simulink library "plant_cl"  (R2018a)
settings: Solver=VariableStepAuto  StartTime=0.0  StopTime=10.0  RelTol=1e-3
undefined symbols (not defined in the file or in its folder): env, faults, p, plant
libraries: lowLevel x29, controllerComponents x1
settings Model: Creator=mitch  LastModifiedBy=mitch

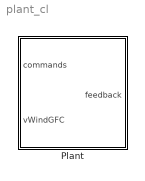
== system plant_cl ==
  Plant : Subsystem

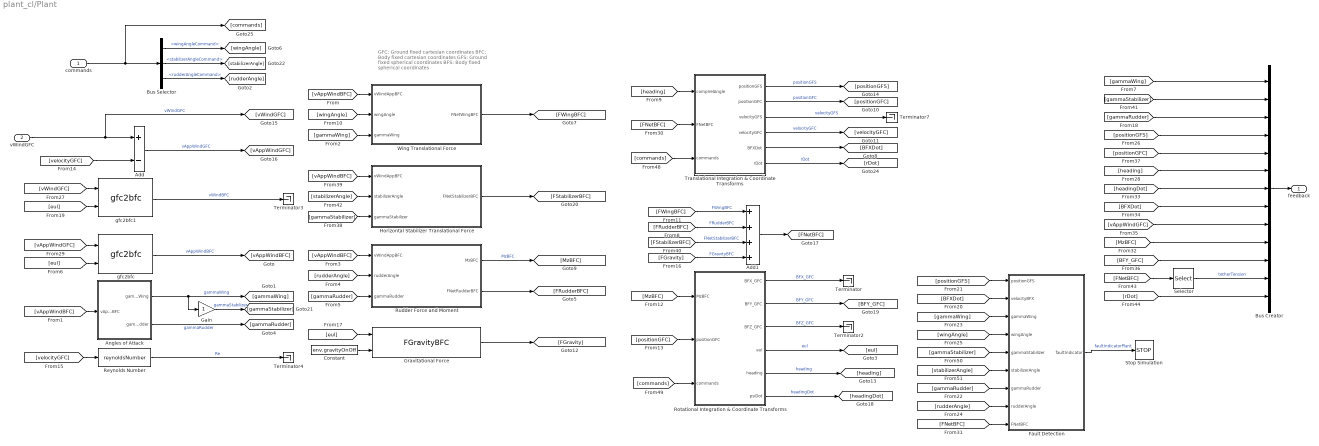
== system plant_cl/Plant ==
  note: GFC: Ground fixed cartesian coordinates
      | BFC:  Body fixed cartesian coordinates
      | GFS: Ground fixed spherical coordinates
      | BFS: Body fixed spherical coordinates
  commands : Inport  OutDataTypeStr=Bus: busControllerOutput
  vWindGFC : Inport  Port=2
  Add : Sum  Inputs=+-
  Add1 : Sum  Inputs=++++
  Angles of Attack : Subsystem
  Bus Selector : BusSelector  OutputSignals=wingAngleCommand,stabilizerAngleCommand,rudderAngleCommand
  Bus Creator : BusCreator  Inputs=13  OutDataTypeStr=Bus: busPlantFeedback
  Constant : Constant  Value=env.gravityOnOff
  Fault Detection : Subsystem
  Gain : Gain
  Gravitational Force : lowLevel/FGravityBFC
  Horizontal Stabilizer Translational Force : Subsystem
  Reynolds Number : lowLevel/reynoldsNumber
  Rotational Integration & Coordinate Transforms : Subsystem
  Rudder Force and Moment : Subsystem
  Selector : Selector  InputPortWidth=3  IndexOptions=Index vector (dialog)  Indices=3  OutputSizes=1
  Stop Simulation : Stop
  Terminator{,2..4,7} (5 alike) : Terminator
  Translational Integration & Coordinate Transforms : Subsystem
  Wing Translational Force : Subsystem
  gfc2bfc : lowLevel/gfc2bfc
  gfc2bfc1 : lowLevel/gfc2bfc
  feedback : Outport  OutDataTypeStr=Bus: busPlantFeedback
  wires:
  vWindGFC/1 -> [vWindGFC], Add/1  "vWindGFC"
  [vAppWindBFC] -> Angles of Attack/1(vAppWindBFC)
  Angles of Attack/1(gammaWing) -> Gain/1, [gammaWing]  "gammaWing"
  [vAppWindBFC] -> Wing Translational Force/1(vWindAppBFC)
  Add/1 -> [vAppWindGFC]  "vAppWindGFC"
  [vAppWindBFC] -> Rudder Force and Moment/1(vWindAppBFC)
  [rudderAngle] -> Rudder Force and Moment/2(rudderAngle)
  Translational Integration & Coordinate Transforms/2(positionGFC) -> [positionGFC]  "positionGFC"
  Rudder Force and Moment/2(FNetRudderBFC) -> [FRudderBFC]
  [gammaWing] -> Wing Translational Force/3(gammaWing)
  [heading] -> Translational Integration & Coordinate Transforms/1(compVelAngle)
  Angles of Attack/2(gammaRudder) -> [gammaRudder]  "gammaRudder"
  [gammaRudder] -> Rudder Force and Moment/3(gammaRudder)
  Wing Translational Force/1(FNetWingBFC) -> [FWingBFC]
  [wingAngle] -> Wing Translational Force/2(wingAngle)
  [FNetBFC] -> Translational Integration & Coordinate Transforms/2(FNetBFC)
  Rudder Force and Moment/1(MzBFC) -> [MzBFC]  "MzBFC"
  [MzBFC] -> Rotational Integration & Coordinate Transforms/1(MzBFC)
  [positionGFC] -> Rotational Integration & Coordinate Transforms/2(positionGFC)
  Rotational Integration & Coordinate Transforms/4(eul) -> [eul]  "eul"
  Rotational Integration & Coordinate Transforms/1(BFX_GFC) -> Terminator/1  "BFX_GFC"
  Rotational Integration & Coordinate Transforms/2(BFY_GFC) -> [BFY_GFC]  "BFY_GFC"
  Rotational Integration & Coordinate Transforms/3(BFZ_GFC) -> Terminator2/1  "BFZ_GFC"
  Translational Integration & Coordinate Transforms/4(velocityGFC) -> [velocityGFC]  "velocityGFC"
  [velocityGFC] -> Add/2
  [velocityGFC] -> Reynolds Number/1
  Reynolds Number/1 -> Terminator4/1  "Re"
  Gravitational Force/1 -> [FGravity]
  [eul] -> Gravitational Force/1
  Translational Integration & Coordinate Transforms/1(positionGFS) -> [positionGFS]  "positionGFS"
  Translational Integration & Coordinate Transforms/3(velocityGFS) -> Terminator7/1  "velocityGFS"
  [eul] -> gfc2bfc1/2
  gfc2bfc1/1 -> Terminator3/1  "vWindBFC"
  Rotational Integration & Coordinate Transforms/5(heading) -> [heading]  "heading"
  Constant/1 -> Gravitational Force/2
  Translational Integration & Coordinate Transforms/5(BFXDot) -> [BFXDot]
  [BFXDot] -> Fault Detection/2(velocityBFX)
  [positionGFS] -> Fault Detection/1(positionGFS)
  Fault Detection/1(faultIndicator) -> Stop Simulation/1  "faultIndicatorPlant"
  [gammaRudder] -> Fault Detection/7(gammaRudder)
  [gammaWing] -> Fault Detection/3(gammaWing)
  [rudderAngle] -> Fault Detection/8(rudderAngle)
  [wingAngle] -> Fault Detection/4(wingAngle)
  [vWindGFC] -> gfc2bfc1/1
  gfc2bfc/1 -> [vAppWindBFC]  "vAppWindBFC"
  [eul] -> gfc2bfc/2
  [vAppWindGFC] -> gfc2bfc/1
  [FWingBFC] -> Add1/1  "FWingBFC"
  [FRudderBFC] -> Add1/2  "FRudderBFC"
  Add1/1 -> [FNetBFC]
  [FNetBFC] -> Fault Detection/9(FNetBFC)
  commands/1 -> [commands], Bus Selector/1
  Bus Selector/1 -> [wingAngle]  "<wingAngleCommand>"
  Bus Selector/3 -> [rudderAngle]  "<rudderAngleCommand>"
  Bus Creator/1 -> feedback/1
  Rotational Integration & Coordinate Transforms/6(psiDot) -> [headingDot]  "headingDot"
  [gammaStabilizer] -> Horizontal Stabilizer Translational Force/3(gammaStabilizer)
  [vAppWindBFC] -> Horizontal Stabilizer Translational Force/1(vWindAppBFC)
  Horizontal Stabilizer Translational Force/1(FNetStabilizerBFC) -> [FStabilizerBFC]
  [FStabilizerBFC] -> Add1/3  "FNetStabilizerBFC"
  [FGravity] -> Add1/4  "FGravityBFC"
  Translational Integration & Coordinate Transforms/6(rDot) -> [rDot]  "rDot"
  [commands] -> Translational Integration & Coordinate Transforms/3(commands)
  [commands] -> Rotational Integration & Coordinate Transforms/3(commands)
  [stabilizerAngle] -> Horizontal Stabilizer Translational Force/2(stabilizerAngle)
  Bus Selector/2 -> [stabilizerAngle]  "<stabilizerAngleCommand>"
  [gammaStabilizer] -> Fault Detection/5(gammaStabilizer)
  [stabilizerAngle] -> Fault Detection/6(stabilizerAngle)
  [gammaWing] -> Bus Creator/1
  [gammaRudder] -> Bus Creator/3
  [rDot] -> Bus Creator/13
  Selector/1 -> Bus Creator/12  "tetherTension"
  [BFY_GFC] -> Bus Creator/11
  [MzBFC] -> Bus Creator/10
  [vAppWindGFC] -> Bus Creator/9
  [BFXDot] -> Bus Creator/8
  [headingDot] -> Bus Creator/7
  [heading] -> Bus Creator/6
  [positionGFC] -> Bus Creator/5
  [positionGFS] -> Bus Creator/4
  [gammaStabilizer] -> Bus Creator/2
  Gain/1 -> [gammaStabilizer]  "gammaStabilizer"
  [FNetBFC] -> Selector/1

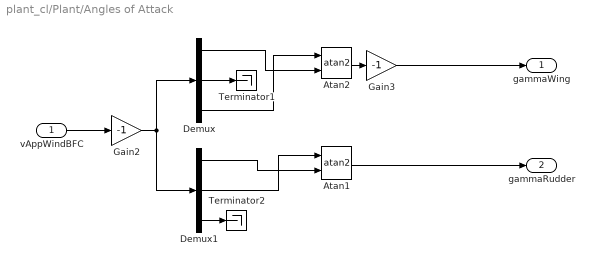
== system plant_cl/Plant/Angles of Attack ==
  vAppWindBFC : Inport
  Atan1 : Trigonometry  Operator=atan2
  Atan2 : Trigonometry  Operator=atan2
  Demux : Demux  Outputs=3
  Demux1 : Demux  Outputs=3
  Gain2 : Gain  Gain=-1
  Gain3 : Gain  Gain=-1
  Terminator1 : Terminator
  Terminator2 : Terminator
  gammaWing : Outport
  gammaRudder : Outport  Port=2
  wires:
  vAppWindBFC/1 -> Gain2/1
  Demux/1 -> Atan2/2
  Atan2/1 -> Gain3/1
  Demux/3 -> Atan2/1
  Demux/2 -> Terminator1/1
  Demux1/3 -> Terminator2/1
  Gain2/1 -> Demux1/1, Demux/1
  Atan1/1 -> gammaRudder/1
  Gain3/1 -> gammaWing/1
  Demux1/1 -> Atan1/2
  Demux1/2 -> Atan1/1

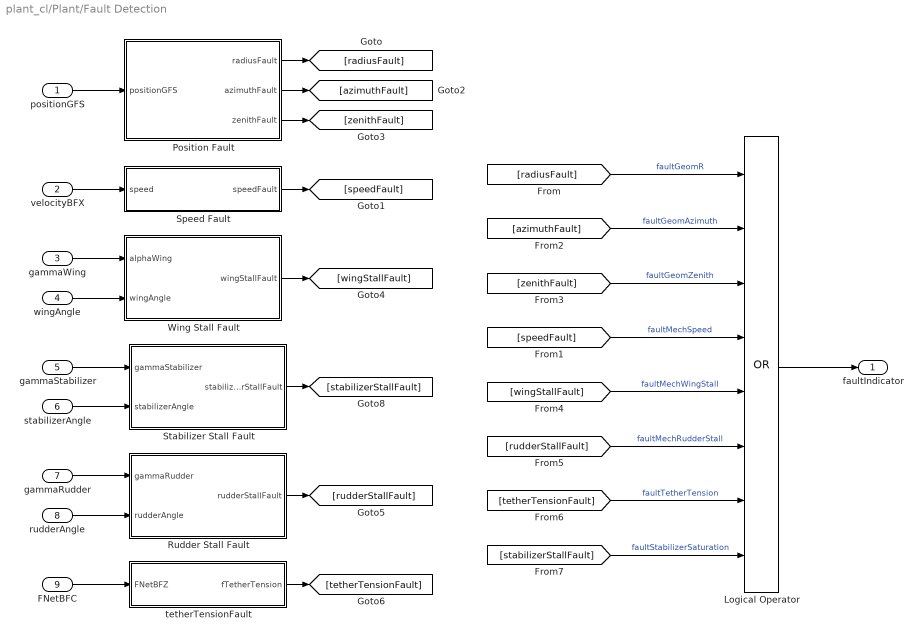
== system plant_cl/Plant/Fault Detection ==
  positionGFS : Inport
  velocityBFX : Inport  Port=2
  gammaWing : Inport  Port=3
  wingAngle : Inport  Port=4
  gammaStabilizer : Inport  Port=5
  stabilizerAngle : Inport  Port=6
  gammaRudder : Inport  Port=7
  rudderAngle : Inport  Port=8
  FNetBFC : Inport  Port=9
  Logical Operator : Logic  Operator=OR  Inputs=8  AllPortsSameDT=off  OutDataTypeStr=boolean
  Position Fault : Subsystem
  Rudder Stall Fault : Subsystem
  Speed Fault : Subsystem
  Stabilizer Stall Fault : Subsystem
  Wing Stall Fault : Subsystem
  tetherTensionFault : Subsystem
  faultIndicator : Outport
  wires:
  positionGFS/1 -> Position Fault/1(positionGFS)
  Logical Operator/1 -> faultIndicator/1
  Speed Fault/1(speedFault) -> [speedFault]
  velocityBFX/1 -> Speed Fault/1(speed)
  [radiusFault] -> Logical Operator/1  "faultGeomR"
  [speedFault] -> Logical Operator/4  "faultMechSpeed"
  [azimuthFault] -> Logical Operator/2  "faultGeomAzimuth"
  [zenithFault] -> Logical Operator/3  "faultGeomZenith"
  Wing Stall Fault/1(wingStallFault) -> [wingStallFault]
  gammaWing/1 -> Wing Stall Fault/1(alphaWing)
  gammaRudder/1 -> Rudder Stall Fault/1(gammaRudder)
  [wingStallFault] -> Logical Operator/5  "faultMechWingStall"
  [rudderStallFault] -> Logical Operator/6  "faultMechRudderStall"
  wingAngle/1 -> Wing Stall Fault/2(wingAngle)
  rudderAngle/1 -> Rudder Stall Fault/2(rudderAngle)
  Rudder Stall Fault/1(rudderStallFault) -> [rudderStallFault]
  Position Fault/1(radiusFault) -> [radiusFault]
  Position Fault/2(azimuthFault) -> [azimuthFault]
  Position Fault/3(zenithFault) -> [zenithFault]
  tetherTensionFault/1(fTetherTension) -> [tetherTensionFault]
  FNetBFC/1 -> tetherTensionFault/1(FNetBFZ)
  [tetherTensionFault] -> Logical Operator/7  "faultTetherTension"
  [stabilizerStallFault] -> Logical Operator/8  "faultStabilizerSaturation"
  gammaStabilizer/1 -> Stabilizer Stall Fault/1(gammaStabilizer)
  Stabilizer Stall Fault/1(stabilizerStallFault) -> [stabilizerStallFault]
  stabilizerAngle/1 -> Stabilizer Stall Fault/2(stabilizerAngle)

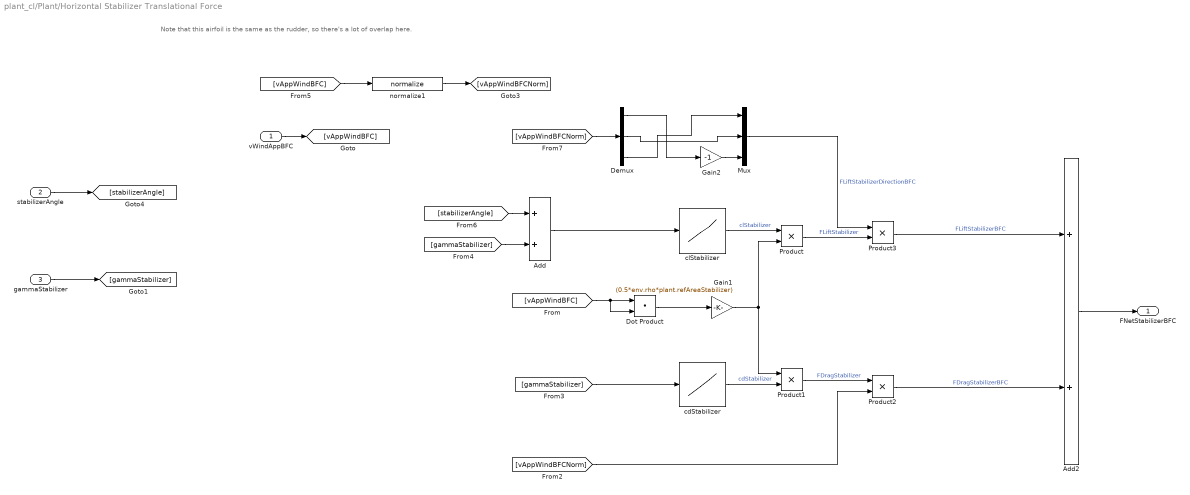
== system plant_cl/Plant/Horizontal Stabilizer Translational Force ==
  note: Note that this airfoil is the same as the rudder, so there's a lot of overlap here.
  vWindAppBFC : Inport
  stabilizerAngle : Inport  Port=2
  gammaStabilizer : Inport  Port=3
  Add : Sum
  Add2 : Sum
  Demux : Demux  Outputs=3
  Dot Product : DotProduct  InputSameDT=on  OutDataTypeStr=Inherit: Inherit via internal rule
  Gain1 : Gain  Gain=(0.5*env.rho*plant.refAreaStabilizer)
  Gain2 : Gain  Gain=-1
  Mux : Mux  Inputs=3
  Product{,1..3} (4 alike) : Product
  cdStabilizer : Lookup_n-D  NumberOfTableDimensions=1  BreakpointsForDimension1=plant.stabilizerTable.alpha  Table=plant.rudderTable.cd  ExtrapMethod=Clip  UseLastTableValue=on  InternalRulePriority=Speed  RndMeth=Simplest  InputSameDT=on
  clStabilizer : Lookup_n-D  NumberOfTableDimensions=1  BreakpointsForDimension1=plant.stabilizerTable.alpha  Table=plant.rudderTable.cl  ExtrapMethod=Clip  UseLastTableValue=on  InternalRulePriority=Speed  RndMeth=Simplest  InputSameDT=on
  normalize1 : lowLevel/normalize
  FNetStabilizerBFC : Outport
  wires:
  Product1/1 -> Product2/1  "FDragStabilizer"
  Product2/1 -> Add2/2  "FDragStabilizerBFC"
  Product/1 -> Product3/2  "FLiftStabilizer"
  Product3/1 -> Add2/1  "FLiftStabilizerBFC"
  Dot Product/1 -> Gain1/1
  clStabilizer/1 -> Product/1  "clStabilizer"
  [vAppWindBFC] -> Dot Product/1, Dot Product/2
  Gain1/1 -> Product/2, Product1/1
  cdStabilizer/1 -> Product1/2  "cdStabilizer"
  vWindAppBFC/1 -> [vAppWindBFC]
  Demux/2 -> Mux/2
  Demux/1 -> Gain2/1
  Mux/1 -> Product3/1  "FLiftStabilizerDirectionBFC"
  Demux/3 -> Mux/1
  [vAppWindBFC] -> normalize1/1
  normalize1/1 -> [vAppWindBFCNorm]
  [vAppWindBFCNorm] -> Demux/1
  [vAppWindBFCNorm] -> Product2/2
  Gain2/1 -> Mux/3
  [gammaStabilizer] -> cdStabilizer/1
  gammaStabilizer/1 -> [gammaStabilizer]
  Add2/1 -> FNetStabilizerBFC/1
  Add/1 -> clStabilizer/1
  [gammaStabilizer] -> Add/2
  stabilizerAngle/1 -> [stabilizerAngle]
  [stabilizerAngle] -> Add/1

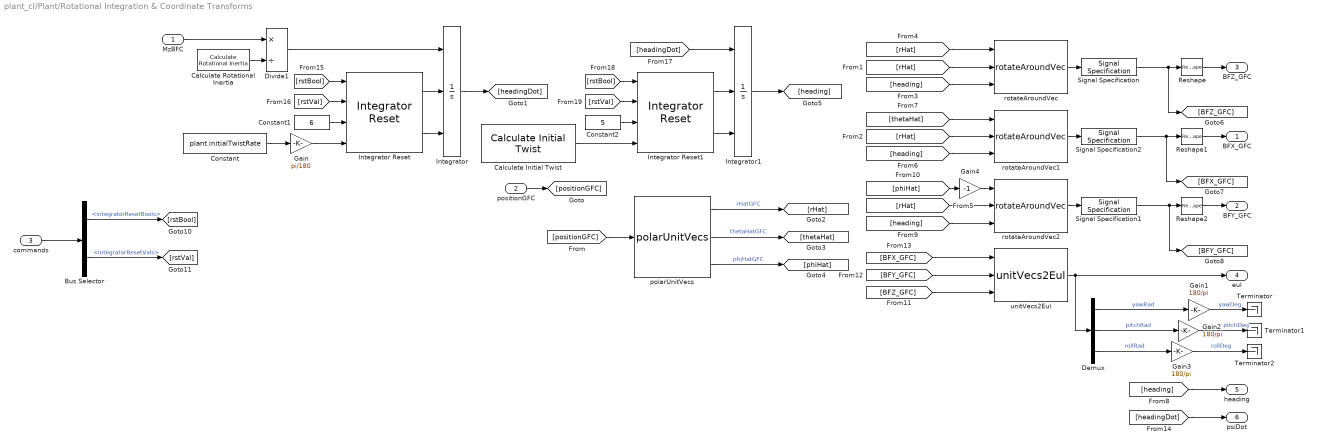
== system plant_cl/Plant/Rotational Integration & Coordinate Transforms ==
  MzBFC : Inport  PortDimensions=1
  positionGFC : Inport  Port=2
  commands : Inport  Port=3  OutDataTypeStr=Bus: busControllerOutput  PortDimensions=1
  Bus Selector : BusSelector  OutputSignals=integratorResetBools,integratorResetVals
  Calculate Rotational Inertia : lowLevel/Calculate Rotational Inertia
  Calculate Initial Twist : controllerComponents/Calculate Initial Twist
  Constant : Constant  Value=plant.initialTwistRate
  Constant1 : Constant  Value=6
  Constant2 : Constant  Value=5
  Demux : Demux  Outputs=3
  Divide1 : Product  Inputs=*/
  Gain : Gain  Gain=pi/180
  Gain1 : Gain  Gain=180/pi
  Gain2 : Gain  Gain=180/pi
  Gain3 : Gain  Gain=180/pi
  Gain4 : Gain  Gain=-1
  Integrator : Integrator  ExternalReset=rising  InitialConditionSource=external  InitialCondition=plant.initialTwistRate
  Integrator Reset : lowLevel/Integrator Reset
  Integrator Reset1 : lowLevel/Integrator Reset
  Integrator1 : Integrator  ExternalReset=rising  InitialConditionSource=external  InitialCondition=plant.initialTwist
  Reshape : Reshape  OutputDimensions=[3 1]
  Reshape1 : Reshape  OutputDimensions=[3 1]
  Reshape2 : Reshape  OutputDimensions=[3 1]
  Signal Specification : SignalSpecification  Dimensions=[1 3]
  Signal Specification1 : SignalSpecification  Dimensions=[1 3]
  Signal Specification2 : SignalSpecification  Dimensions=[1 3]
  Terminator : Terminator
  Terminator1 : Terminator
  Terminator2 : Terminator
  polarUnitVecs : lowLevel/polarUnitVecs
  rotateAroundVec : lowLevel/rotateAroundVec
  rotateAroundVec1 : lowLevel/rotateAroundVec
  rotateAroundVec2 : lowLevel/rotateAroundVec
  unitVecs2Eul : lowLevel/unitVecs2Eul
  BFX_GFC : Outport
  BFY_GFC : Outport  Port=2
  BFZ_GFC : Outport  Port=3
  eul : Outport  Port=4  PortDimensions=3
  heading : Outport  Port=5  PortDimensions=1
  psiDot : Outport  Port=6  PortDimensions=1
  wires:
  MzBFC/1 -> Divide1/1
  Integrator/1 -> [headingDot]
  positionGFC/1 -> [positionGFC]
  [positionGFC] -> polarUnitVecs/1
  polarUnitVecs/1 -> [rHat]  "rHatGFC"
  polarUnitVecs/2 -> [thetaHat]  "thetaHatGFC"
  polarUnitVecs/3 -> [phiHat]  "phiHatGFC"
  Integrator1/1 -> [heading]
  [heading] -> rotateAroundVec/3
  [rHat] -> rotateAroundVec/1
  [rHat] -> rotateAroundVec/2
  [thetaHat] -> rotateAroundVec1/1
  [heading] -> rotateAroundVec1/3
  [rHat] -> rotateAroundVec1/2
  [phiHat] -> Gain4/1
  [heading] -> rotateAroundVec2/3
  [rHat] -> rotateAroundVec2/2
  unitVecs2Eul/1 -> Demux/1, eul/1
  [BFZ_GFC] -> unitVecs2Eul/3
  [BFY_GFC] -> unitVecs2Eul/2
  [BFX_GFC] -> unitVecs2Eul/1
  Demux/3 -> Gain3/1  "rollRad"
  Demux/2 -> Gain2/1  "pitchRad"
  Demux/1 -> Gain1/1  "yawRad"
  Gain1/1 -> Terminator/1  "yawDeg"
  Gain2/1 -> Terminator1/1  "pitchDeg"
  Gain3/1 -> Terminator2/1  "rollDeg"
  Gain4/1 -> rotateAroundVec2/1
  rotateAroundVec/1 -> Signal Specification/1
  rotateAroundVec1/1 -> Signal Specification2/1
  rotateAroundVec2/1 -> Signal Specification1/1
  Signal Specification/1 -> Reshape/1, [BFZ_GFC]
  Signal Specification2/1 -> [BFX_GFC], Reshape1/1
  Signal Specification1/1 -> [BFY_GFC], Reshape2/1
  Reshape/1 -> BFZ_GFC/1
  Reshape1/1 -> BFX_GFC/1
  Reshape2/1 -> BFY_GFC/1
  [heading] -> heading/1
  [headingDot] -> psiDot/1
  Calculate Rotational Inertia/1 -> Divide1/2
  Divide1/1 -> Integrator/1
  Bus Selector/2 -> [rstVal]  "<integratorResetVals>"
  commands/1 -> Bus Selector/1
  Bus Selector/1 -> [rstBool]  "<integratorResetBools>"
  Integrator Reset1/1 -> Integrator1/2
  Integrator Reset1/2 -> Integrator1/3
  Integrator Reset/1 -> Integrator/2
  Integrator Reset/2 -> Integrator/3
  Constant/1 -> Gain/1
  [rstBool] -> Integrator Reset/1
  [rstVal] -> Integrator Reset/2
  Constant1/1 -> Integrator Reset/3
  Gain/1 -> Integrator Reset/4
  [headingDot] -> Integrator1/1
  [rstVal] -> Integrator Reset1/2
  Constant2/1 -> Integrator Reset1/3
  [rstBool] -> Integrator Reset1/1
  Calculate Initial Twist/1 -> Integrator Reset1/4

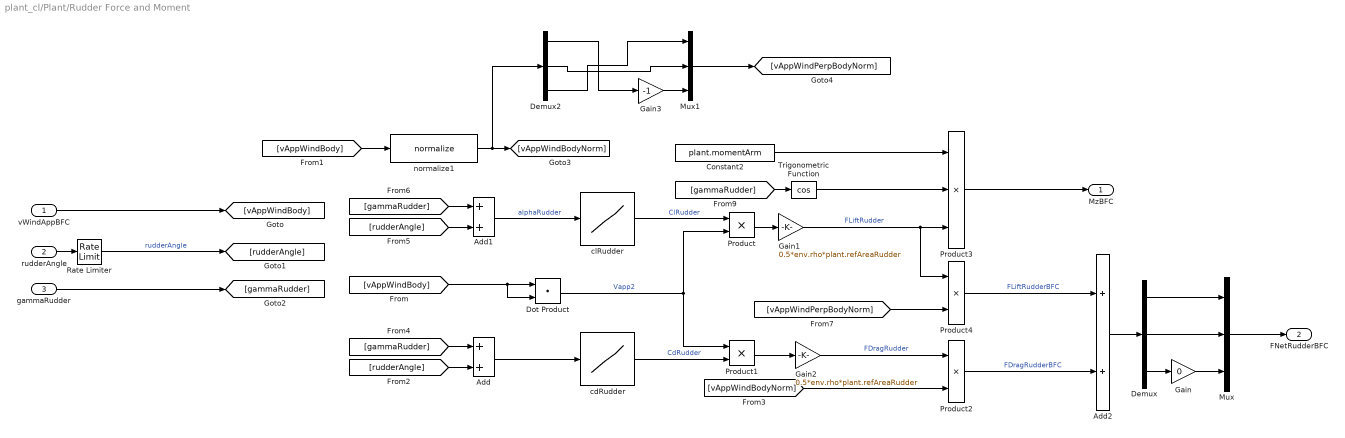
== system plant_cl/Plant/Rudder Force and Moment ==
  vWindAppBFC : Inport
  rudderAngle : Inport  Port=2
  gammaRudder : Inport  Port=3
  Add : Sum
  Add1 : Sum
  Add2 : Sum
  Constant2 : Constant  Value=plant.momentArm
  Demux : Demux  Outputs=3
  Demux2 : Demux  Outputs=3
  Dot Product : DotProduct  InputSameDT=on  OutDataTypeStr=Inherit: Inherit via internal rule
  Gain : Gain  Gain=0
  Gain1 : Gain  Gain=0.5*env.rho*plant.refAreaRudder
  Gain2 : Gain  Gain=0.5*env.rho*plant.refAreaRudder
  Gain3 : Gain  Gain=-1
  Mux : Mux  Inputs=3
  Mux1 : Mux  Inputs=3
  Product{,1..2,4} (4 alike) : Product
  Product3 : Product  Inputs=3
  Rate Limiter : RateLimiter  RisingSlewLimit=plant.rudderAngleRateLimit*pi/180  FallingSlewLimit=-plant.rudderAngleRateLimit*pi/180  SampleTimeMode=inherited
  Trigonometric Function : Trigonometry  Operator=cos
  cdRudder : Lookup_n-D  NumberOfTableDimensions=1  BreakpointsForDimension1=plant.rudderTable.alpha  Table=plant.rudderTable.cd  ExtrapMethod=Clip  UseLastTableValue=on  InternalRulePriority=Speed  RndMeth=Simplest  InputSameDT=on
  clRudder : Lookup_n-D  NumberOfTableDimensions=1  BreakpointsForDimension1=plant.rudderTable.alpha  Table=plant.rudderTable.cl  ExtrapMethod=Clip  UseLastTableValue=on  InternalRulePriority=Speed  RndMeth=Simplest  InputSameDT=on
  normalize1 : lowLevel/normalize
  MzBFC : Outport
  FNetRudderBFC : Outport  Port=2
  wires:
  clRudder/1 -> Product/1  "ClRudder"
  [vAppWindBody] -> Dot Product/2, Dot Product/1
  Dot Product/1 -> Product1/1, Product/2  "Vapp2"
  vWindAppBFC/1 -> [vAppWindBody]
  rudderAngle/1 -> Rate Limiter/1
  Product/1 -> Gain1/1
  cdRudder/1 -> Product1/2  "CdRudder"
  Product1/1 -> Gain2/1
  Gain2/1 -> Product2/1  "FDragRudder"
  [vAppWindBodyNorm] -> Product2/2
  gammaRudder/1 -> [gammaRudder]
  [rudderAngle] -> Add/2
  [gammaRudder] -> Add/1
  Add/1 -> cdRudder/1
  [rudderAngle] -> Add1/2
  [gammaRudder] -> Add1/1
  Add1/1 -> clRudder/1  "alphaRudder"
  Gain1/1 -> Product4/1, Product3/3  "FLiftRudder"
  [vAppWindBody] -> normalize1/1
  Rate Limiter/1 -> [rudderAngle]  "rudderAngle"
  Product2/1 -> Add2/2  "FDragRudderBFC"
  [gammaRudder] -> Trigonometric Function/1
  Trigonometric Function/1 -> Product3/2
  Constant2/1 -> Product3/1
  Product3/1 -> MzBFC/1
  Product4/1 -> Add2/1  "FLiftRudderBFC"
  Mux/1 -> FNetRudderBFC/1
  Add2/1 -> Demux/1
  Demux/2 -> Mux/2
  Demux/1 -> Mux/1
  Demux/3 -> Gain/1
  Gain/1 -> Mux/3
  Demux2/2 -> Mux1/2
  Gain3/1 -> Mux1/3
  normalize1/1 -> Demux2/1, [vAppWindBodyNorm]
  Demux2/1 -> Gain3/1
  Demux2/3 -> Mux1/1
  Mux1/1 -> [vAppWindPerpBodyNorm]
  [vAppWindPerpBodyNorm] -> Product4/2

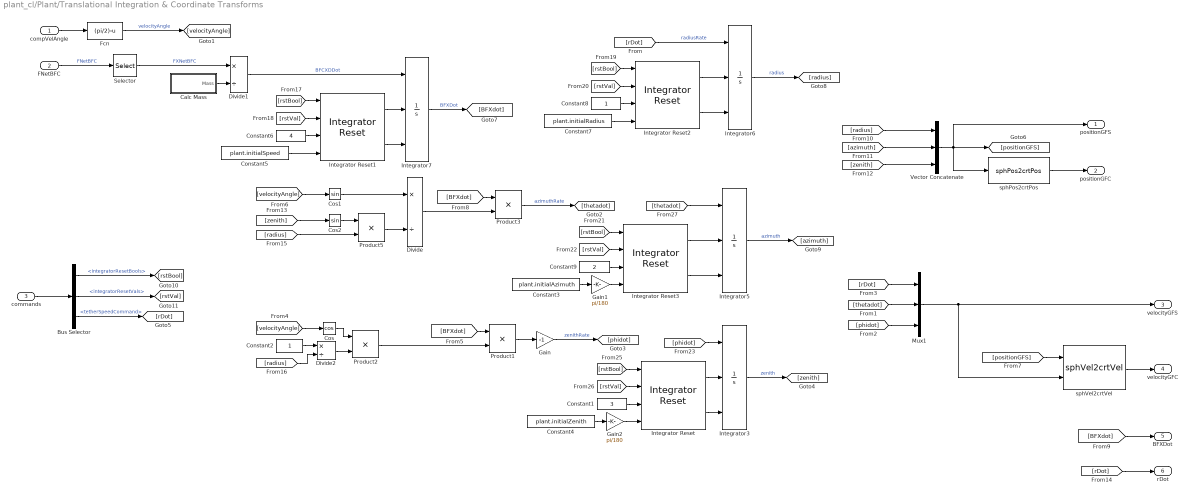
== system plant_cl/Plant/Translational Integration & Coordinate Transforms ==
  compVelAngle : Inport
  FNetBFC : Inport  Port=2
  commands : Inport  Port=3  OutDataTypeStr=Bus: busControllerOutput
  Bus Selector : BusSelector  OutputSignals=integratorResetBools,integratorResetVals,tetherSpeedCommand
  Calc Mass : Subsystem
  Constant1 : Constant  Value=3
  Constant2 : Constant
  Constant3 : Constant  Value=plant.initialAzimuth
  Constant4 : Constant  Value=plant.initialZenith
  Constant5 : Constant  Value=plant.initialSpeed
  Constant6 : Constant  Value=4
  Constant7 : Constant  Value=plant.initialRadius
  Constant8 : Constant
  Constant9 : Constant  Value=2
  Cos : Trigonometry  Operator=cos
  Cos1 : Trigonometry
  Cos2 : Trigonometry
  Divide : Product  Inputs=*/
  Divide1 : Product  Inputs=*/
  Divide2 : Product  Inputs=*/
  Fcn : Fcn  Expr=(pi/2)-u
  Gain : Gain  Gain=-1
  Gain1 : Gain  Gain=pi/180
  Gain2 : Gain  Gain=pi/180
  Integrator Reset{,1..3} (4 alike) : lowLevel/Integrator Reset
  Integrator3 : Integrator  ExternalReset=rising  InitialConditionSource=external  InitialCondition=p.initPositionGFS(3)
  Integrator5 : Integrator  ExternalReset=rising  InitialConditionSource=external  InitialCondition=p.initPositionGFS(2)
  Integrator6 : Integrator  ExternalReset=rising  InitialConditionSource=external  InitialCondition=p.initPositionGFS(1)
  Integrator7 : Integrator  ExternalReset=rising  InitialConditionSource=external  InitialCondition=p.initVelocity
  Mux1 : Mux  Inputs=3
  Product{1..3,5} (4 alike) : Product
  Selector : Selector  InputPortWidth=3  IndexOptions=Index vector (dialog)  Indices=1  OutputSizes=1
  Vector Concatenate : Concatenate  NumInputs=3
  sphPos2crtPos : lowLevel/sphPos2crtPos
  sphVel2crtVel : lowLevel/sphVel2crtVel
  positionGFS : Outport  PortDimensions=3
  positionGFC : Outport  Port=2  PortDimensions=3
  velocityGFS : Outport  Port=3  PortDimensions=3
  velocityGFC : Outport  Port=4  PortDimensions=3
  BFXDot : Outport  Port=5
  rDot : Outport  Port=6
  wires:
  Gain/1 -> [phidot]  "zenithRate"
  Integrator5/1 -> [azimuth]  "azimuth"
  Product3/1 -> [thetadot]  "azimuthRate"
  Integrator3/1 -> [zenith]  "zenith"
  sphPos2crtPos/1 -> positionGFC/1
  sphVel2crtVel/1 -> velocityGFC/1
  [rDot] -> Mux1/1
  [thetadot] -> Mux1/2
  [phidot] -> Mux1/3
  FNetBFC/1 -> Selector/1  "FNetBFC"
  compVelAngle/1 -> Fcn/1
  Integrator6/1 -> [radius]  "radius"
  Mux1/1 -> sphVel2crtVel/2, velocityGFS/1
  [rDot] -> Integrator6/1  "radiusRate"
  [positionGFS] -> sphVel2crtVel/1
  Fcn/1 -> [velocityAngle]  "velocityAngle"
  [BFXdot] -> Product3/1
  [velocityAngle] -> Cos1/1
  Divide/1 -> Product3/2
  Cos1/1 -> Divide/1
  [radius] -> Product5/2
  [zenith] -> Cos2/1
  Cos2/1 -> Product5/1
  Product5/1 -> Divide/2
  [BFXdot] -> Product1/1
  [velocityAngle] -> Cos/1
  Product2/1 -> Product1/2
  Cos/1 -> Product2/1
  Divide2/1 -> Product2/2
  Product1/1 -> Gain/1
  Integrator7/1 -> [BFXdot]  "BFXDot"
  Divide1/1 -> Integrator7/1  "BFCXDDot"
  [BFXdot] -> BFXDot/1
  Vector Concatenate/1 -> [positionGFS], positionGFS/1, sphPos2crtPos/1
  [radius] -> Vector Concatenate/1
  [azimuth] -> Vector Concatenate/2
  [zenith] -> Vector Concatenate/3
  Selector/1 -> Divide1/1  "FXNetBFC"
  Calc Mass/1(Mass) -> Divide1/2
  [rDot] -> rDot/1
  [radius] -> Divide2/2
  Constant2/1 -> Divide2/1
  commands/1 -> Bus Selector/1
  Bus Selector/1 -> [rstBool]  "<integratorResetBools>"
  Bus Selector/2 -> [rstVal]  "<integratorResetVals>"
  Integrator Reset1/1 -> Integrator7/2
  Integrator Reset2/2 -> Integrator6/3
  Integrator Reset1/2 -> Integrator7/3
  Integrator Reset3/1 -> Integrator5/2
  Integrator Reset3/2 -> Integrator5/3
  Integrator Reset2/1 -> Integrator6/2
  [rstBool] -> Integrator Reset/1
  [rstVal] -> Integrator Reset/2
  Constant1/1 -> Integrator Reset/3
  Constant3/1 -> Gain1/1
  Constant4/1 -> Gain2/1
  [rstVal] -> Integrator Reset1/2
  [rstBool] -> Integrator Reset1/1
  Constant6/1 -> Integrator Reset1/3
  Constant5/1 -> Integrator Reset1/4
  [rstVal] -> Integrator Reset2/2
  [rstBool] -> Integrator Reset2/1
  Constant8/1 -> Integrator Reset2/3
  Bus Selector/3 -> [rDot]  "<tetherSpeedCommand>"
  Constant7/1 -> Integrator Reset2/4
  [rstVal] -> Integrator Reset3/2
  [rstBool] -> Integrator Reset3/1
  Constant9/1 -> Integrator Reset3/3
  Gain1/1 -> Integrator Reset3/4
  [thetadot] -> Integrator5/1
  Gain2/1 -> Integrator Reset/4
  Integrator Reset/1 -> Integrator3/2
  Integrator Reset/2 -> Integrator3/3
  [phidot] -> Integrator3/1

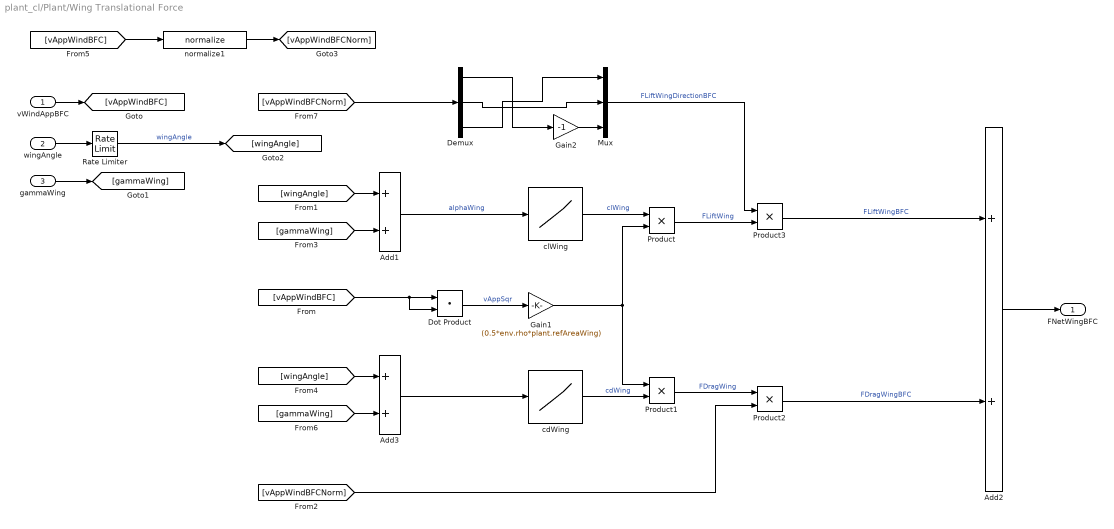
== system plant_cl/Plant/Wing Translational Force ==
  vWindAppBFC : Inport
  wingAngle : Inport  Port=2
  gammaWing : Inport  Port=3
  Add1 : Sum
  Add2 : Sum
  Add3 : Sum
  Demux : Demux  Outputs=3
  Dot Product : DotProduct  InputSameDT=on  OutDataTypeStr=Inherit: Inherit via internal rule
  Gain1 : Gain  Gain=(0.5*env.rho*plant.refAreaWing)
  Gain2 : Gain  Gain=-1
  Mux : Mux  Inputs=3
  Product{,1..3} (4 alike) : Product
  Rate Limiter : RateLimiter  RisingSlewLimit=plant.wingAngleRateLimit*pi/180  FallingSlewLimit=-plant.wingAngleRateLimit*pi/180  SampleTimeMode=inherited
  cdWing : Lookup_n-D  NumberOfTableDimensions=1  BreakpointsForDimension1=plant.wingTable.alpha  Table=plant.wingTable.cd  ExtrapMethod=Clip  UseLastTableValue=on  InternalRulePriority=Speed  RndMeth=Simplest  InputSameDT=on
  clWing : Lookup_n-D  NumberOfTableDimensions=1  BreakpointsForDimension1=plant.wingTable.alpha  Table=plant.wingTable.cl  ExtrapMethod=Clip  UseLastTableValue=on  InternalRulePriority=Speed  RndMeth=Simplest  InputSameDT=on
  normalize1 : lowLevel/normalize
  FNetWingBFC : Outport
  wires:
  Product1/1 -> Product2/1  "FDragWing"
  Product2/1 -> Add2/2  "FDragWingBFC"
  Product/1 -> Product3/2  "FLiftWing"
  Product3/1 -> Add2/1  "FLiftWingBFC"
  Dot Product/1 -> Gain1/1  "vAppSqr"
  clWing/1 -> Product/1  "clWing"
  [vAppWindBFC] -> Dot Product/2, Dot Product/1
  Gain1/1 -> Product/2, Product1/1
  cdWing/1 -> Product1/2  "cdWing"
  vWindAppBFC/1 -> [vAppWindBFC]
  Add2/1 -> FNetWingBFC/1
  gammaWing/1 -> [gammaWing]
  wingAngle/1 -> Rate Limiter/1
  [wingAngle] -> Add3/1
  [gammaWing] -> Add3/2
  Demux/1 -> Gain2/1
  Mux/1 -> Product3/1  "FLiftWingDirectionBFC"
  Demux/3 -> Mux/1
  [vAppWindBFC] -> normalize1/1
  normalize1/1 -> [vAppWindBFCNorm]
  [vAppWindBFCNorm] -> Demux/1
  [vAppWindBFCNorm] -> Product2/2
  Gain2/1 -> Mux/3
  Add3/1 -> cdWing/1
  [wingAngle] -> Add1/1
  [gammaWing] -> Add1/2
  Add1/1 -> clWing/1  "alphaWing"
  Rate Limiter/1 -> [wingAngle]  "wingAngle"
  Demux/2 -> Mux/2

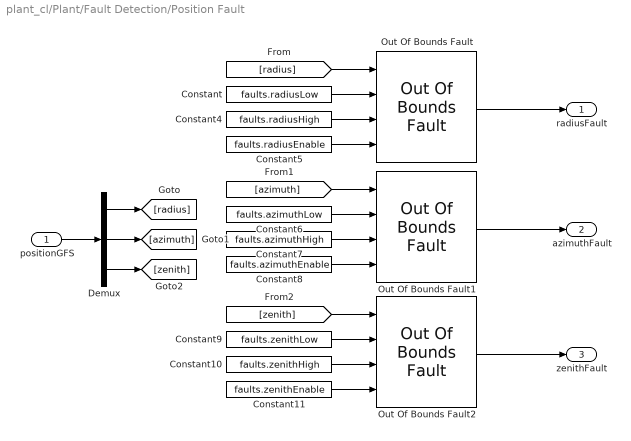
== system plant_cl/Plant/Fault Detection/Position Fault ==
  positionGFS : Inport
  Constant : Constant  Value=faults.radiusLow
  Constant10 : Constant  Value=faults.zenithHigh
  Constant11 : Constant  Value=faults.zenithEnable
  Constant4 : Constant  Value=faults.radiusHigh
  Constant5 : Constant  Value=faults.radiusEnable
  Constant6 : Constant  Value=faults.azimuthLow
  Constant7 : Constant  Value=faults.azimuthHigh
  Constant8 : Constant  Value=faults.azimuthEnable
  Constant9 : Constant  Value=faults.zenithLow
  Demux : Demux  Outputs=3
  Out Of Bounds Fault : lowLevel/Out Of Bounds Fault
  Out Of Bounds Fault1 : lowLevel/Out Of Bounds Fault
  Out Of Bounds Fault2 : lowLevel/Out Of Bounds Fault
  radiusFault : Outport
  azimuthFault : Outport  Port=2
  zenithFault : Outport  Port=3
  wires:
  positionGFS/1 -> Demux/1
  Out Of Bounds Fault/1 -> radiusFault/1
  Out Of Bounds Fault1/1 -> azimuthFault/1
  Out Of Bounds Fault2/1 -> zenithFault/1
  Demux/1 -> [radius]
  Demux/2 -> [azimuth]
  Demux/3 -> [zenith]
  [radius] -> Out Of Bounds Fault/1
  [azimuth] -> Out Of Bounds Fault1/1
  [zenith] -> Out Of Bounds Fault2/1
  Constant/1 -> Out Of Bounds Fault/2
  Constant5/1 -> Out Of Bounds Fault/4
  Constant4/1 -> Out Of Bounds Fault/3
  Constant7/1 -> Out Of Bounds Fault1/3
  Constant6/1 -> Out Of Bounds Fault1/2
  Constant8/1 -> Out Of Bounds Fault1/4
  Constant9/1 -> Out Of Bounds Fault2/2
  Constant10/1 -> Out Of Bounds Fault2/3
  Constant11/1 -> Out Of Bounds Fault2/4

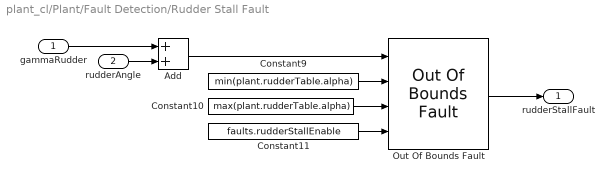
== system plant_cl/Plant/Fault Detection/Rudder Stall Fault ==
  gammaRudder : Inport
  rudderAngle : Inport  Port=2
  Add : Sum
  Constant10 : Constant  Value=max(plant.rudderTable.alpha)
  Constant11 : Constant  Value=faults.rudderStallEnable
  Constant9 : Constant  Value=min(plant.rudderTable.alpha)
  Out Of Bounds Fault : lowLevel/Out Of Bounds Fault
  rudderStallFault : Outport
  wires:
  rudderAngle/1 -> Add/2
  gammaRudder/1 -> Add/1
  Out Of Bounds Fault/1 -> rudderStallFault/1
  Constant9/1 -> Out Of Bounds Fault/2
  Constant11/1 -> Out Of Bounds Fault/4
  Constant10/1 -> Out Of Bounds Fault/3
  Add/1 -> Out Of Bounds Fault/1

== system plant_cl/Plant/Fault Detection/Speed Fault ==
  note: If body fixed speed in x is negative
  speed : Inport
  Constant10 : Constant  Value=faults.speedHigh
  Constant11 : Constant  Value=faults.speedEnable
  Constant9 : Constant  Value=faults.speedLow
  Out Of Bounds Fault : lowLevel/Out Of Bounds Fault
  speedFault : Outport
  wires:
  speed/1 -> Out Of Bounds Fault/1
  Constant9/1 -> Out Of Bounds Fault/2
  Constant10/1 -> Out Of Bounds Fault/3
  Constant11/1 -> Out Of Bounds Fault/4
  Out Of Bounds Fault/1 -> speedFault/1

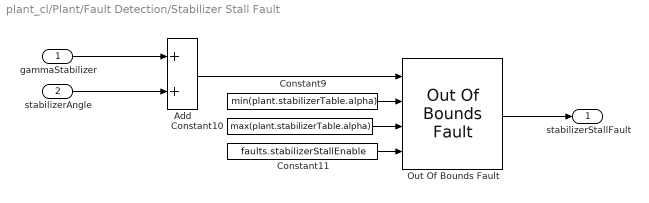
== system plant_cl/Plant/Fault Detection/Stabilizer Stall Fault ==
  gammaStabilizer : Inport
  stabilizerAngle : Inport  Port=2
  Add : Sum
  Constant10 : Constant  Value=max(plant.stabilizerTable.alpha)
  Constant11 : Constant  Value=faults.stabilizerStallEnable
  Constant9 : Constant  Value=min(plant.stabilizerTable.alpha)
  Out Of Bounds Fault : lowLevel/Out Of Bounds Fault
  stabilizerStallFault : Outport
  wires:
  Out Of Bounds Fault/1 -> stabilizerStallFault/1
  Constant10/1 -> Out Of Bounds Fault/3
  Constant11/1 -> Out Of Bounds Fault/4
  Constant9/1 -> Out Of Bounds Fault/2
  gammaStabilizer/1 -> Add/1
  stabilizerAngle/1 -> Add/2
  Add/1 -> Out Of Bounds Fault/1

== system plant_cl/Plant/Fault Detection/Wing Stall Fault ==
  alphaWing : Inport
  wingAngle : Inport  Port=2
  Add : Sum
  Constant10 : Constant  Value=max(plant.wingTable.alpha)
  Constant11 : Constant  Value=faults.wingStallEnable
  Constant9 : Constant  Value=min(plant.wingTable.alpha)
  Out Of Bounds Fault : lowLevel/Out Of Bounds Fault
  wingStallFault : Outport
  wires:
  alphaWing/1 -> Add/1
  wingAngle/1 -> Add/2
  Out Of Bounds Fault/1 -> wingStallFault/1
  Constant11/1 -> Out Of Bounds Fault/4
  Constant10/1 -> Out Of Bounds Fault/3
  Constant9/1 -> Out Of Bounds Fault/2
  Add/1 -> Out Of Bounds Fault/1

== system plant_cl/Plant/Fault Detection/tetherTensionFault ==
  note: If net force in body fixed Z direction is zero or negative
  FNetBFZ : Inport
  Constant10 : Constant  Value=faults.tetherTensionHigh
  Constant11 : Constant  Value=faults.tetherTensionEnable
  Constant9 : Constant  Value=faults.tetherTensionLow
  Out Of Bounds Fault : lowLevel/Out Of Bounds Fault
  Selector : Selector  InputPortWidth=3  IndexOptions=Index vector (dialog)  Indices=3  OutputSizes=1
  fTetherTension : Outport
  wires:
  FNetBFZ/1 -> Selector/1
  Selector/1 -> Out Of Bounds Fault/1
  Constant9/1 -> Out Of Bounds Fault/2
  Constant10/1 -> Out Of Bounds Fault/3
  Constant11/1 -> Out Of Bounds Fault/4
  Out Of Bounds Fault/1 -> fTetherTension/1

== system plant_cl/Plant/Translational Integration & Coordinate Transforms/Calc Mass ==
  Add1 : Sum
  Constant1 : Constant  Value=plant.addedMassMultiplier
  Constant2 : Constant  Value=plant.mass
  Constant4 : Constant  Value=env.rho
  Product3 : Product
  Mass : Outport
  wires:
  Constant4/1 -> Product3/1
  Add1/1 -> Mass/1
  Product3/1 -> Add1/1
  Constant2/1 -> Add1/2
  Constant1/1 -> Product3/2
